simulink subsystem "Led_Ctrl"  (R2023b)
settings: Solver=VariableStepAuto  StartTime=0.0  StopTime=10.0  RelTol=1e-3
libraries: simulink x1
settings Model: Creator=m4ttn  LastModifiedBy=m4ttn
settings RTWCC: GPUComputeCapability=5.0

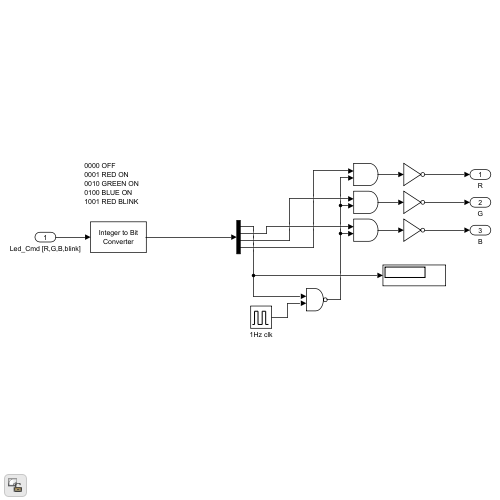
[thumbnail: Simulink's stored preview of the top-level diagram]
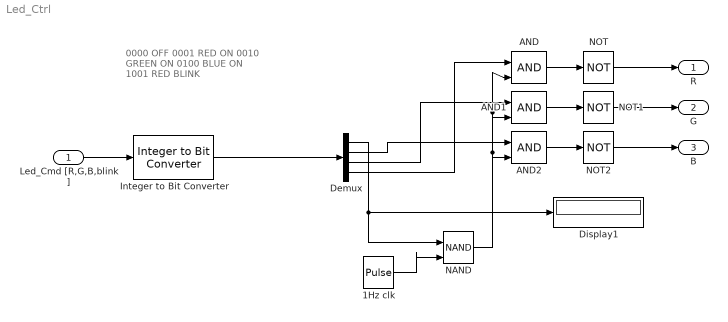
== system Led_Ctrl ==
  note: 0000 OFF
      | 0001 RED ON
      | 0010 GREEN ON
      | 0100 BLUE ON
      | 1001 RED BLINK
  Led_Cmd [R,G,B,blink] : Inport  OutDataTypeStr=uint8
  1Hz clk : DiscretePulseGenerator  PulseType=Time based  Period=1  PulseWidth=50
  AND : Logic  IconShape=distinctive  AllPortsSameDT=off  OutDataTypeStr=boolean
  AND1 : Logic  IconShape=distinctive  AllPortsSameDT=off  OutDataTypeStr=boolean
  AND2 : Logic  IconShape=distinctive  AllPortsSameDT=off  OutDataTypeStr=boolean
  Demux : Demux
  Display1 : Display
  Integer to Bit Converter : simulink/Logic and Bit Operations/Integer to Bit Converter  nbits=4  signedInputValues=Unsigned  bitOrder=MSB first  outDtype=Inherit via internal rule
  NAND : Logic  Operator=NAND  IconShape=distinctive  AllPortsSameDT=off  OutDataTypeStr=boolean
  NOT : Logic  Operator=NOT  IconShape=distinctive  AllPortsSameDT=off  OutDataTypeStr=boolean
  NOT1 : Logic  Operator=NOT  IconShape=distinctive  AllPortsSameDT=off  OutDataTypeStr=boolean
  NOT2 : Logic  Operator=NOT  IconShape=distinctive  AllPortsSameDT=off  OutDataTypeStr=boolean
  R : Outport  OutDataTypeStr=boolean
  G : Outport  Port=2  OutDataTypeStr=boolean
  B : Outport  Port=3  OutDataTypeStr=boolean
  wires:
  Led_Cmd [R,G,B,blink]/1 -> Integer to Bit Converter/1
  1Hz clk/1 -> NAND/2
  NAND/1 -> AND/2, AND1/2, AND2/2
  AND/1 -> NOT/1
  Demux/1 -> NAND/1, Display1/1
  Demux/4 -> AND/1
  Demux/3 -> AND1/1
  Demux/2 -> AND2/1
  Integer to Bit Converter/1 -> Demux/1
  NOT/1 -> R/1
  NOT2/1 -> B/1
  AND2/1 -> NOT2/1
  AND1/1 -> NOT1/1
  NOT1/1 -> G/1
